simulink model "compare"  (R2018b)
settings: Solver=VariableStepAuto  StartTime=0.0  StopTime=10.0  RelTol=1e-3
values from neighbouring files (symbols this model uses):
  x = -10:1:20    [FSK.m]    (also in compare.m = -10:1:15)
undefined symbols (not defined in the file or in its folder): i
libraries: commdigbbndpm3 x4, commchan3 x3, commsink2 x3, commdigbbndfm2 x2, commrandsrc3 x1
settings Model: Creator=Aurora  LastModifiedBy=Aurora

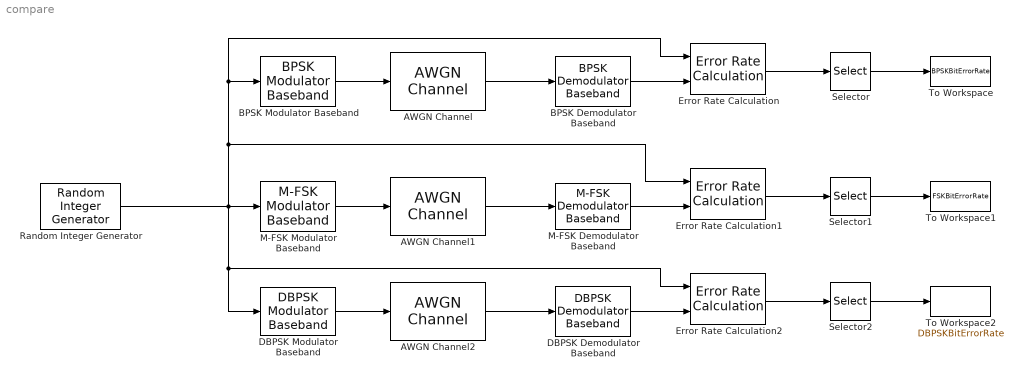
== system compare ==
  AWGN Channel : commchan3/AWGN Channel  InputProcessing=Columns as channels (frame based)  seed=67  noiseMode="Signal to noise ratio  (SNR)"  EbNodB=10  EsNodB=10  SNRdB=x(i)  bitsPerSym=1  Ps=1  Tsym=1  variance=1
  AWGN Channel1 : commchan3/AWGN Channel  InputProcessing=Columns as channels (frame based)  seed=67  noiseMode="Signal to noise ratio  (SNR)"  EbNodB=10  EsNodB=10  SNRdB=x(i)  bitsPerSym=1  Ps=1  Tsym=1  variance=1
  AWGN Channel2 : commchan3/AWGN Channel  InputProcessing=Columns as channels (frame based)  seed=67  noiseMode="Signal to noise ratio  (SNR)"  EbNodB=10  EsNodB=10  SNRdB=x(i)  bitsPerSym=1  Ps=1  Tsym=1  variance=1
  BPSK Demodulator Baseband : commdigbbndpm3/BPSK Demodulator Baseband  DecType=Hard decision  VarSource=Dialog  Variance=1  Ph=pi/8  outDtype=Inherit via internal rule  derotateFactorWordLen=16  derotateFactorDataTypeStr=Inherit: Same word length as input  derotateFactorLastDataTypeStr=Inherit: Same word length as input
  BPSK Modulator Baseband : commdigbbndpm3/BPSK Modulator Baseband  Ph=pi/8  outDtype=double  outWordLen=16  outUDDataType=sfix(16)  outFracLenMode=Best precision  outFracLen=15  outDataTypeStr=double  outLastDataTypeStr=double
  DBPSK Demodulator Baseband : commdigbbndpm3/DBPSK Demodulator Baseband  Ph=pi/8  outDtype=Inherit via internal rule
      settings: SourceProductName=Communications System Toolbox  SourceProductBaseCode=CM
  DBPSK Modulator Baseband : commdigbbndpm3/DBPSK Modulator Baseband  Ph=pi/8  outDtype=double
      settings: SourceProductName=Communications System Toolbox  SourceProductBaseCode=CM
  Error Rate Calculation : commsink2/Error Rate Calculation  N=0  st_delay=0  cp_mode=Entire frame  subframe=[]  PMode=Port  WsName=ErrorVec  RsMode2=off  stop=off  numErr=100  maxBits=1e6
  Error Rate Calculation1 : commsink2/Error Rate Calculation  N=0  st_delay=0  cp_mode=Entire frame  subframe=[]  PMode=Port  WsName=ErrorVec  RsMode2=off  stop=off  numErr=100  maxBits=1e6
  Error Rate Calculation2 : commsink2/Error Rate Calculation  N=0  st_delay=0  cp_mode=Entire frame  subframe=[]  PMode=Port  WsName=ErrorVec  RsMode2=off  stop=off  numErr=100  maxBits=1e6
  M-FSK Demodulator Baseband : commdigbbndfm2/M-FSK Demodulator Baseband  M=2  OutType=Bit  Dec=Binary  freqSep=1000  numSamp=17  RateOptions=Enforce single-rate processing  outDataType=double
      settings: SourceProductName=Communications System Toolbox  SourceProductBaseCode=CM
  M-FSK Modulator Baseband : commdigbbndfm2/M-FSK Modulator Baseband  M=2  InType=Bit  Enc=Binary  freqSep=2000  phaseType=Continuous  numSamp=17  RateOptions=Enforce single-rate processing  outDataType=double
      settings: SourceProductName=Communications System Toolbox
  Random Integer Generator : commrandsrc3/Random Integer Generator  SetSize=2  SeedSource=Parameter  Seed=37  SampleTime=0.0001  SamplesPerFrame=10000  OutputDataType=double  SimulateUsing=Interpreted execution
  Selector : Selector  InputPortWidth=3  IndexOptions=Index vector (dialog)  Indices=[1]  OutputSizes=1
  Selector1 : Selector  InputPortWidth=3  IndexOptions=Index vector (dialog)  Indices=[1]  OutputSizes=1
  Selector2 : Selector  InputPortWidth=3  IndexOptions=Index vector (dialog)  Indices=[1]  OutputSizes=1
  To Workspace : ToWorkspace  VariableName=BPSKBitErrorRate  SampleTime=-1
      settings: Save2DSignal=2-D array (concatenate along first dimension)
  To Workspace1 : ToWorkspace  VariableName=FSKBitErrorRate  SampleTime=-1
      settings: Save2DSignal=2-D array (concatenate along first dimension)
  To Workspace2 : ToWorkspace  VariableName=DBPSKBitErrorRate  SampleTime=-1
      settings: Save2DSignal=2-D array (concatenate along first dimension)
  wires:
  Error Rate Calculation/1 -> Selector/1
  AWGN Channel/1 -> BPSK Demodulator Baseband/1
  BPSK Modulator Baseband/1 -> AWGN Channel/1
  Selector/1 -> To Workspace/1
  Random Integer Generator/1 -> BPSK Modulator Baseband/1, Error Rate Calculation/1, Error Rate Calculation1/1, Error Rate Calculation2/1, DBPSK Modulator Baseband/1, M-FSK Modulator Baseband/1
  BPSK Demodulator Baseband/1 -> Error Rate Calculation/2
  M-FSK Demodulator Baseband/1 -> Error Rate Calculation1/2
  AWGN Channel1/1 -> M-FSK Demodulator Baseband/1
  Error Rate Calculation1/1 -> Selector1/1
  Selector1/1 -> To Workspace1/1
  M-FSK Modulator Baseband/1 -> AWGN Channel1/1
  DBPSK Demodulator Baseband/1 -> Error Rate Calculation2/2
  AWGN Channel2/1 -> DBPSK Demodulator Baseband/1
  Error Rate Calculation2/1 -> Selector2/1
  Selector2/1 -> To Workspace2/1
  DBPSK Modulator Baseband/1 -> AWGN Channel2/1
